simulink model "quadsim"  (R2021a)
settings: Solver=ode45  StartTime=0.0  StopTime=20  FixedStep=0.001  RelTol=1e-3  EnableMultiTasking=on
InitFcn:
  | param
undefined symbols (not defined in the file or in its folder): controller, P, trajectory
settings Model: NumberOfSteps=100  Creator=ecestudent  LastModifiedBy=ncrl
settings SolverCC: AlgebraicLoopSolver=TrustRegion
settings DataIOCC: LimitDataPoints=on  SaveFormat=Array  ReturnWorkspaceOutputs=off
settings OptimizationCC: LifeSpan=inf
settings DebuggingCC: SFUnexpectedBacktrackingDiag=warning  SFNoUnconditionalDefaultTransitionDiag=warning  SFExecutionAtInitializationDiag=none  SFMachineParentedDataDiag=warning  ArithmeticOperatorsInVariantConditions=warning
settings HardwareCC: ProdBitPerPointer=32  ProdBitPerSizeT=32  ProdBitPerPtrDiffT=32  ProdLargestAtomicFloat=None  ProdIntDivRoundTo=Undefined  ProdEndianess=Unspecified  ProdWordSize=32  ProdHWDeviceType=32-bit Generic
settings ModelReferenceCC: PropagateSignalLabelsOutOfModel=off
settings SFSimCC: SimUseLocalCustomCode=off  CustomCodeUndefinedFunction=UseInterfaceOnly
settings RTWCC: RTWUseLocalCustomCode=off
settings CodeAppCC: StateflowObjectComments=on
settings GRTTargetCC: TargetLangStandard=C89/C90 (ANSI)
settings ConfigComp: CovMetricSettings=dw  CovSaveCumulativeToWorkspaceVar=on  CovSaveSingleToWorkspaceVar=on  CovExternalEMLEnable=off
settings SimscapeCC: SimscapeNormalizeSystem=off

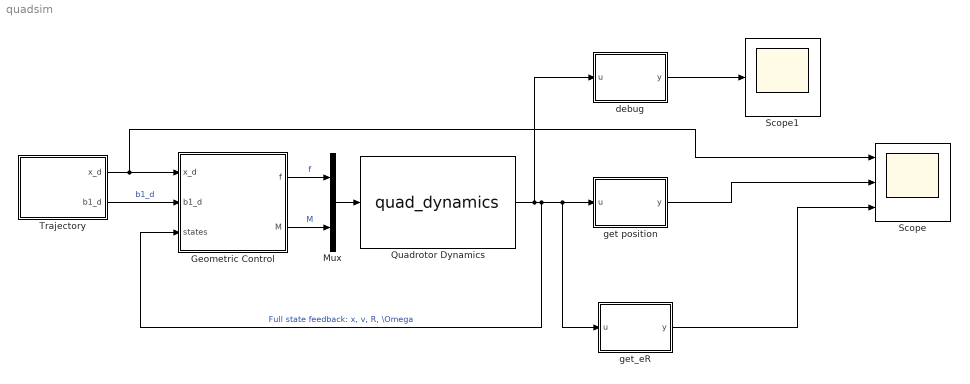
== system quadsim ==
  Geometric Control : Subsystem
  Mux : Mux  Inputs=2
  Quadrotor Dynamics : S-Function  FunctionName=quad_dynamics  Parameters=P  SFunctionDeploymentMode=off  EnableBusSupport=off
  Scope : Scope  NumInputPorts=3
  Scope1 : Scope
  Trajectory : Subsystem
  debug : MATLAB Function  TreatAsAtomicUnit=on
  get position : MATLAB Function  TreatAsAtomicUnit=on
  get_eR : MATLAB Function  TreatAsAtomicUnit=on
  wires:
  Mux/1 -> Quadrotor Dynamics/1
  Quadrotor Dynamics/1 -> debug/1(u), get_eR/1(u), get position/1(u), Geometric Control/3(states)  "Full state feedback: x, v, R, \\Omega"
  Geometric Control/1(f) -> Mux/1  "f"
  Geometric Control/2(M) -> Mux/2  "M"
  Trajectory/1(x_d) -> Scope/1, Geometric Control/1(x_d)
  Trajectory/2(b1_d) -> Geometric Control/2(b1_d)  "b1_d"
  get position/1(y) -> Scope/2
  get_eR/1(y) -> Scope/3
  debug/1(y) -> Scope1/1

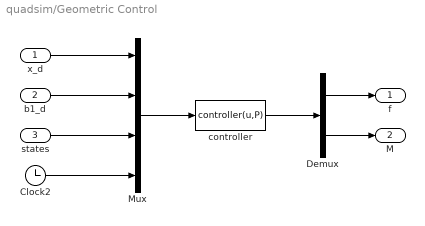
== system quadsim/Geometric Control ==
  x_d : Inport
  b1_d : Inport  Port=2
  states : Inport  Port=3
  Clock2 : Clock
  Demux : Demux  Outputs=2
  Mux : Mux
  controller : MATLABFcn  MATLABFcn=controller(u,P)  OutputDimensions=4  SampleTime=P.Ts
  f : Outport  VectorParamsAs1DForOutWhenUnconnected=off
  M : Outport  Port=2  VectorParamsAs1DForOutWhenUnconnected=off
  wires:
  Clock2/1 -> Mux/4
  Mux/1 -> controller/1
  x_d/1 -> Mux/1
  states/1 -> Mux/3
  Demux/1 -> f/1
  Demux/2 -> M/1
  b1_d/1 -> Mux/2
  controller/1 -> Demux/1

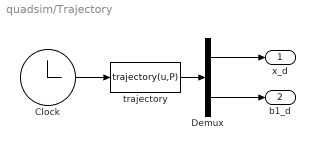
== system quadsim/Trajectory ==
  Clock : Clock
  Demux : Demux  Outputs=2
  trajectory : MATLABFcn  MATLABFcn=trajectory(u,P)  OutputDimensions=6
  x_d : Outport  VectorParamsAs1DForOutWhenUnconnected=off
  b1_d : Outport  Port=2  VectorParamsAs1DForOutWhenUnconnected=off
  wires:
  Clock/1 -> trajectory/1
  trajectory/1 -> Demux/1
  Demux/1 -> x_d/1
  Demux/2 -> b1_d/1

== matlab function quadsim/get position ==
  data: u input; y output
function y = fcn(u)

y = u(1:3);
end

== matlab function quadsim/debug ==
  data: u input; y output
function y = fcn(u)


R     = reshape(u(7:15),3,3);
y = R;
end

== matlab function quadsim/get_eR ==
  data: u input; y output
function y = get_eR(u)

R  = reshape(u(7:15),3,3);
Rd = [1 0 0; 0 1 0; 0 0 1];
eR = 0.5 * vee(Rd' * R - R' * Rd);
y = eR;

end
